simulink model "hip_controller_2026_01_27"  (R2024b)
settings: Solver=FixedStepAuto  StartTime=0.0  StopTime=simDuration  FixedStep=0.01  RelTol=1e-3  EnableMultiTasking=on
InitFcn:
  | breakp=[-1, -0.8, -0.6, -0.4, -0.2, -0.1, 0, 0.1, 0.2, 0.4, 0.6, 0.8, 1];
  | splinenew =[-1, -0.8, -0.6, -0.4, -0.2, -0.1, 0, 0, 0.005, 0.01, 0.015,0.02,0.025];
undefined symbols (not defined in the file or in its folder): Discrete, K, qbreak, Time
libraries: simulink x53, arduinolib x11, dspswit3 x9, ctrlSharedLib x2, dspfdesign x2, slpidlib x2
(part 4 of 4)

== system hip_controller_2026_01_27/Subsystem3/Right Motor Velocity/Subsystem/CAN Pack1/Subsystem/Buff 2 ==
  In1 : Inport
  Constant2 : Constant  Value=4  OutDataTypeStr=uint16
  Data Type Conversion2 : DataTypeConversion  OutDataTypeStr=uint8  SaturateOnIntegerOverflow=off  RndMeth=Floor
  Shift Arithmetic1 : ArithShift  BitShiftNumberSource=Input port  BitShiftNumber=8  BitShiftDirection=Right
      settings: InputPortMap=u0,p1
  Out1 : Outport
  wires:
  Shift Arithmetic1/1 -> Data Type Conversion2/1
  Data Type Conversion2/1 -> Out1/1
  In1/1 -> Shift Arithmetic1/1
  Constant2/1 -> Shift Arithmetic1/2

== system hip_controller_2026_01_27/Subsystem3/Right Motor Velocity/Subsystem/CAN Pack1/Subsystem/Buff 3 ==
  In1 : Inport
  In2 : Inport  Port=2
  Bitwise AND1 : simulink/Logic and Bit Operations/Bitwise Operator  logicop=AND  UseBitMask=on  BitMask=bin2dec('000000001111')  BitMaskRealWorld=Stored Integer
  Bitwise OR1 : simulink/Logic and Bit Operations/Bitwise Operator  logicop=OR  UseBitMask=off  NumInputPorts=2  BitMask=bin2dec('11011001')  BitMaskRealWorld=Stored Integer
  Constant1 : Constant  Value=8  OutDataTypeStr=uint16
  Constant2 : Constant  Value=4  OutDataTypeStr=uint16
  Data Type Conversion3 : DataTypeConversion  OutDataTypeStr=uint8  SaturateOnIntegerOverflow=off  RndMeth=Floor
  Shift Arithmetic3 : ArithShift  BitShiftNumberSource=Input port  BitShiftNumber=8  BitShiftDirection=Left
      settings: InputPortMap=u0,p1
  Shift Arithmetic4 : ArithShift  BitShiftNumberSource=Input port  BitShiftNumber=8  BitShiftDirection=Right
      settings: InputPortMap=u0,p1
  Out1 : Outport
  wires:
  Shift Arithmetic3/1 -> Bitwise OR1/1
  In1/1 -> Bitwise AND1/1
  Constant1/1 -> Shift Arithmetic4/2
  Bitwise AND1/1 -> Shift Arithmetic3/1
  Shift Arithmetic4/1 -> Bitwise OR1/2
  In2/1 -> Shift Arithmetic4/1
  Bitwise OR1/1 -> Data Type Conversion3/1
  Data Type Conversion3/1 -> Out1/1
  Constant2/1 -> Shift Arithmetic3/2

== system hip_controller_2026_01_27/Subsystem3/Right Motor Velocity/Subsystem/CAN Pack1/Subsystem/Buff 4 ==
  In1 : Inport
  Bitwise AND3 : simulink/Logic and Bit Operations/Bitwise Operator  logicop=AND  UseBitMask=on  BitMask=bin2dec('000011111111')  BitMaskRealWorld=Stored Integer
  Data Type Conversion4 : DataTypeConversion  OutDataTypeStr=uint8  SaturateOnIntegerOverflow=off  RndMeth=Floor
  Out1 : Outport
  wires:
  Data Type Conversion4/1 -> Out1/1
  Bitwise AND3/1 -> Data Type Conversion4/1
  In1/1 -> Bitwise AND3/1

== system hip_controller_2026_01_27/Subsystem3/Right Motor Velocity/Subsystem/CAN Pack1/Subsystem/Buff 5 ==
  In2 : Inport
  Constant2 : Constant  Value=4  OutDataTypeStr=uint16
  Data Type Conversion5 : DataTypeConversion  OutDataTypeStr=uint8  SaturateOnIntegerOverflow=off  RndMeth=Floor
  Shift Arithmetic5 : ArithShift  BitShiftNumberSource=Input port  BitShiftNumber=8  BitShiftDirection=Right
      settings: InputPortMap=u0,p1
  Out1 : Outport
  wires:
  In2/1 -> Shift Arithmetic5/1
  Shift Arithmetic5/1 -> Data Type Conversion5/1
  Data Type Conversion5/1 -> Out1/1
  Constant2/1 -> Shift Arithmetic5/2

== system hip_controller_2026_01_27/Subsystem3/Right Motor Velocity/Subsystem/CAN Pack1/Subsystem/Buff 6 ==
  In3 : Inport
  In4 : Inport  Port=2
  Bitwise AND2 : simulink/Logic and Bit Operations/Bitwise Operator  logicop=AND  UseBitMask=on  BitMask=bin2dec('000000001111')  BitMaskRealWorld=Stored Integer
  Bitwise OR2 : simulink/Logic and Bit Operations/Bitwise Operator  logicop=OR  UseBitMask=off  NumInputPorts=2  BitMask=bin2dec('11011001')  BitMaskRealWorld=Stored Integer
  Constant1 : Constant  Value=8  OutDataTypeStr=uint16
  Constant2 : Constant  Value=4  OutDataTypeStr=uint16
  Data Type Conversion6 : DataTypeConversion  OutDataTypeStr=uint8  SaturateOnIntegerOverflow=off  RndMeth=Floor
  Shift Arithmetic6 : ArithShift  BitShiftNumberSource=Input port  BitShiftNumber=8  BitShiftDirection=Left
      settings: InputPortMap=u0,p1
  Shift Arithmetic7 : ArithShift  BitShiftNumberSource=Input port  BitShiftNumber=8  BitShiftDirection=Right
      settings: InputPortMap=u0,p1
  Out1 : Outport
  wires:
  In4/1 -> Shift Arithmetic7/1
  Shift Arithmetic7/1 -> Bitwise OR2/2
  Shift Arithmetic6/1 -> Bitwise OR2/1
  Bitwise OR2/1 -> Data Type Conversion6/1
  In3/1 -> Bitwise AND2/1
  Bitwise AND2/1 -> Shift Arithmetic6/1
  Data Type Conversion6/1 -> Out1/1
  Constant2/1 -> Shift Arithmetic6/2
  Constant1/1 -> Shift Arithmetic7/2

== system hip_controller_2026_01_27/Subsystem3/Right Motor Velocity/Subsystem/CAN Pack1/Subsystem/Buff 7 ==
  In1 : Inport
  Bitwise AND4 : simulink/Logic and Bit Operations/Bitwise Operator  logicop=AND  UseBitMask=on  BitMask=bin2dec('000011111111')  BitMaskRealWorld=Stored Integer
  Data Type Conversion7 : DataTypeConversion  OutDataTypeStr=uint8  SaturateOnIntegerOverflow=off  RndMeth=Floor
  Out1 : Outport
  wires:
  Bitwise AND4/1 -> Data Type Conversion7/1
  Data Type Conversion7/1 -> Out1/1
  In1/1 -> Bitwise AND4/1

== system hip_controller_2026_01_27/Subsystem4/Left Motor Velocity/Subsystem/CAN Pack1/Subsystem/Buff 0 ==
  In1 : Inport
  Constant1 : Constant  Value=8  OutDataTypeStr=uint16
  Data Type Conversion : DataTypeConversion  OutDataTypeStr=uint8  SaturateOnIntegerOverflow=off  RndMeth=Floor
  Shift Arithmetic2 : ArithShift  BitShiftNumberSource=Input port  BitShiftNumber=8  BitShiftDirection=Right
      settings: InputPortMap=u0,p1
  Out1 : Outport
  wires:
  In1/1 -> Shift Arithmetic2/1
  Shift Arithmetic2/1 -> Data Type Conversion/1
  Data Type Conversion/1 -> Out1/1
  Constant1/1 -> Shift Arithmetic2/2

== system hip_controller_2026_01_27/Subsystem4/Left Motor Velocity/Subsystem/CAN Pack1/Subsystem/Buff 1 ==
  In1 : Inport
  Bitwise AND : simulink/Logic and Bit Operations/Bitwise Operator  logicop=AND  UseBitMask=on  BitMask=bin2dec('0000000011111111')  BitMaskRealWorld=Stored Integer
  Data Type Conversion1 : DataTypeConversion  OutDataTypeStr=uint8  SaturateOnIntegerOverflow=off  RndMeth=Floor
  Out1 : Outport
  wires:
  Bitwise AND/1 -> Data Type Conversion1/1
  Data Type Conversion1/1 -> Out1/1
  In1/1 -> Bitwise AND/1

== system hip_controller_2026_01_27/Subsystem4/Left Motor Velocity/Subsystem/CAN Pack1/Subsystem/Buff 2 ==
  In1 : Inport
  Constant2 : Constant  Value=4  OutDataTypeStr=uint16
  Data Type Conversion2 : DataTypeConversion  OutDataTypeStr=uint8  SaturateOnIntegerOverflow=off  RndMeth=Floor
  Shift Arithmetic1 : ArithShift  BitShiftNumberSource=Input port  BitShiftNumber=8  BitShiftDirection=Right
      settings: InputPortMap=u0,p1
  Out1 : Outport
  wires:
  Shift Arithmetic1/1 -> Data Type Conversion2/1
  Data Type Conversion2/1 -> Out1/1
  In1/1 -> Shift Arithmetic1/1
  Constant2/1 -> Shift Arithmetic1/2

== system hip_controller_2026_01_27/Subsystem4/Left Motor Velocity/Subsystem/CAN Pack1/Subsystem/Buff 3 ==
  In1 : Inport
  In2 : Inport  Port=2
  Bitwise AND1 : simulink/Logic and Bit Operations/Bitwise Operator  logicop=AND  UseBitMask=on  BitMask=bin2dec('000000001111')  BitMaskRealWorld=Stored Integer
  Bitwise OR1 : simulink/Logic and Bit Operations/Bitwise Operator  logicop=OR  UseBitMask=off  NumInputPorts=2  BitMask=bin2dec('11011001')  BitMaskRealWorld=Stored Integer
  Constant1 : Constant  Value=8  OutDataTypeStr=uint16
  Constant2 : Constant  Value=4  OutDataTypeStr=uint16
  Data Type Conversion3 : DataTypeConversion  OutDataTypeStr=uint8  SaturateOnIntegerOverflow=off  RndMeth=Floor
  Shift Arithmetic3 : ArithShift  BitShiftNumberSource=Input port  BitShiftNumber=8  BitShiftDirection=Left
      settings: InputPortMap=u0,p1
  Shift Arithmetic4 : ArithShift  BitShiftNumberSource=Input port  BitShiftNumber=8  BitShiftDirection=Right
      settings: InputPortMap=u0,p1
  Out1 : Outport
  wires:
  Shift Arithmetic3/1 -> Bitwise OR1/1
  In1/1 -> Bitwise AND1/1
  Constant1/1 -> Shift Arithmetic4/2
  Bitwise AND1/1 -> Shift Arithmetic3/1
  Shift Arithmetic4/1 -> Bitwise OR1/2
  In2/1 -> Shift Arithmetic4/1
  Bitwise OR1/1 -> Data Type Conversion3/1
  Data Type Conversion3/1 -> Out1/1
  Constant2/1 -> Shift Arithmetic3/2

== system hip_controller_2026_01_27/Subsystem4/Left Motor Velocity/Subsystem/CAN Pack1/Subsystem/Buff 4 ==
  In1 : Inport
  Bitwise AND3 : simulink/Logic and Bit Operations/Bitwise Operator  logicop=AND  UseBitMask=on  BitMask=bin2dec('000011111111')  BitMaskRealWorld=Stored Integer
  Data Type Conversion4 : DataTypeConversion  OutDataTypeStr=uint8  SaturateOnIntegerOverflow=off  RndMeth=Floor
  Out1 : Outport
  wires:
  Data Type Conversion4/1 -> Out1/1
  Bitwise AND3/1 -> Data Type Conversion4/1
  In1/1 -> Bitwise AND3/1

== system hip_controller_2026_01_27/Subsystem4/Left Motor Velocity/Subsystem/CAN Pack1/Subsystem/Buff 5 ==
  In2 : Inport
  Constant2 : Constant  Value=4  OutDataTypeStr=uint16
  Data Type Conversion5 : DataTypeConversion  OutDataTypeStr=uint8  SaturateOnIntegerOverflow=off  RndMeth=Floor
  Shift Arithmetic5 : ArithShift  BitShiftNumberSource=Input port  BitShiftNumber=8  BitShiftDirection=Right
      settings: InputPortMap=u0,p1
  Out1 : Outport
  wires:
  In2/1 -> Shift Arithmetic5/1
  Shift Arithmetic5/1 -> Data Type Conversion5/1
  Data Type Conversion5/1 -> Out1/1
  Constant2/1 -> Shift Arithmetic5/2

== system hip_controller_2026_01_27/Subsystem4/Left Motor Velocity/Subsystem/CAN Pack1/Subsystem/Buff 6 ==
  In3 : Inport
  In4 : Inport  Port=2
  Bitwise AND2 : simulink/Logic and Bit Operations/Bitwise Operator  logicop=AND  UseBitMask=on  BitMask=bin2dec('000000001111')  BitMaskRealWorld=Stored Integer
  Bitwise OR2 : simulink/Logic and Bit Operations/Bitwise Operator  logicop=OR  UseBitMask=off  NumInputPorts=2  BitMask=bin2dec('11011001')  BitMaskRealWorld=Stored Integer
  Constant1 : Constant  Value=8  OutDataTypeStr=uint16
  Constant2 : Constant  Value=4  OutDataTypeStr=uint16
  Data Type Conversion6 : DataTypeConversion  OutDataTypeStr=uint8  SaturateOnIntegerOverflow=off  RndMeth=Floor
  Shift Arithmetic6 : ArithShift  BitShiftNumberSource=Input port  BitShiftNumber=8  BitShiftDirection=Left
      settings: InputPortMap=u0,p1
  Shift Arithmetic7 : ArithShift  BitShiftNumberSource=Input port  BitShiftNumber=8  BitShiftDirection=Right
      settings: InputPortMap=u0,p1
  Out1 : Outport
  wires:
  In4/1 -> Shift Arithmetic7/1
  Shift Arithmetic7/1 -> Bitwise OR2/2
  Shift Arithmetic6/1 -> Bitwise OR2/1
  Bitwise OR2/1 -> Data Type Conversion6/1
  In3/1 -> Bitwise AND2/1
  Bitwise AND2/1 -> Shift Arithmetic6/1
  Data Type Conversion6/1 -> Out1/1
  Constant2/1 -> Shift Arithmetic6/2
  Constant1/1 -> Shift Arithmetic7/2

== system hip_controller_2026_01_27/Subsystem4/Left Motor Velocity/Subsystem/CAN Pack1/Subsystem/Buff 7 ==
  In1 : Inport
  Bitwise AND4 : simulink/Logic and Bit Operations/Bitwise Operator  logicop=AND  UseBitMask=on  BitMask=bin2dec('000011111111')  BitMaskRealWorld=Stored Integer
  Data Type Conversion7 : DataTypeConversion  OutDataTypeStr=uint8  SaturateOnIntegerOverflow=off  RndMeth=Floor
  Out1 : Outport
  wires:
  Bitwise AND4/1 -> Data Type Conversion7/1
  Data Type Conversion7/1 -> Out1/1
  In1/1 -> Bitwise AND4/1

== system hip_controller_2026_01_27/Subsystem4/Right Motor Velocity/Subsystem/CAN Pack1/Subsystem/Buff 0 ==
  In1 : Inport
  Constant1 : Constant  Value=8  OutDataTypeStr=uint16
  Data Type Conversion : DataTypeConversion  OutDataTypeStr=uint8  SaturateOnIntegerOverflow=off  RndMeth=Floor
  Shift Arithmetic2 : ArithShift  BitShiftNumberSource=Input port  BitShiftNumber=8  BitShiftDirection=Right
      settings: InputPortMap=u0,p1
  Out1 : Outport
  wires:
  In1/1 -> Shift Arithmetic2/1
  Shift Arithmetic2/1 -> Data Type Conversion/1
  Data Type Conversion/1 -> Out1/1
  Constant1/1 -> Shift Arithmetic2/2

== system hip_controller_2026_01_27/Subsystem4/Right Motor Velocity/Subsystem/CAN Pack1/Subsystem/Buff 1 ==
  In1 : Inport
  Bitwise AND : simulink/Logic and Bit Operations/Bitwise Operator  logicop=AND  UseBitMask=on  BitMask=bin2dec('0000000011111111')  BitMaskRealWorld=Stored Integer
  Data Type Conversion1 : DataTypeConversion  OutDataTypeStr=uint8  SaturateOnIntegerOverflow=off  RndMeth=Floor
  Out1 : Outport
  wires:
  Bitwise AND/1 -> Data Type Conversion1/1
  Data Type Conversion1/1 -> Out1/1
  In1/1 -> Bitwise AND/1

== system hip_controller_2026_01_27/Subsystem4/Right Motor Velocity/Subsystem/CAN Pack1/Subsystem/Buff 2 ==
  In1 : Inport
  Constant2 : Constant  Value=4  OutDataTypeStr=uint16
  Data Type Conversion2 : DataTypeConversion  OutDataTypeStr=uint8  SaturateOnIntegerOverflow=off  RndMeth=Floor
  Shift Arithmetic1 : ArithShift  BitShiftNumberSource=Input port  BitShiftNumber=8  BitShiftDirection=Right
      settings: InputPortMap=u0,p1
  Out1 : Outport
  wires:
  Shift Arithmetic1/1 -> Data Type Conversion2/1
  Data Type Conversion2/1 -> Out1/1
  In1/1 -> Shift Arithmetic1/1
  Constant2/1 -> Shift Arithmetic1/2

== system hip_controller_2026_01_27/Subsystem4/Right Motor Velocity/Subsystem/CAN Pack1/Subsystem/Buff 3 ==
  In1 : Inport
  In2 : Inport  Port=2
  Bitwise AND1 : simulink/Logic and Bit Operations/Bitwise Operator  logicop=AND  UseBitMask=on  BitMask=bin2dec('000000001111')  BitMaskRealWorld=Stored Integer
  Bitwise OR1 : simulink/Logic and Bit Operations/Bitwise Operator  logicop=OR  UseBitMask=off  NumInputPorts=2  BitMask=bin2dec('11011001')  BitMaskRealWorld=Stored Integer
  Constant1 : Constant  Value=8  OutDataTypeStr=uint16
  Constant2 : Constant  Value=4  OutDataTypeStr=uint16
  Data Type Conversion3 : DataTypeConversion  OutDataTypeStr=uint8  SaturateOnIntegerOverflow=off  RndMeth=Floor
  Shift Arithmetic3 : ArithShift  BitShiftNumberSource=Input port  BitShiftNumber=8  BitShiftDirection=Left
      settings: InputPortMap=u0,p1
  Shift Arithmetic4 : ArithShift  BitShiftNumberSource=Input port  BitShiftNumber=8  BitShiftDirection=Right
      settings: InputPortMap=u0,p1
  Out1 : Outport
  wires:
  Shift Arithmetic3/1 -> Bitwise OR1/1
  In1/1 -> Bitwise AND1/1
  Constant1/1 -> Shift Arithmetic4/2
  Bitwise AND1/1 -> Shift Arithmetic3/1
  Shift Arithmetic4/1 -> Bitwise OR1/2
  In2/1 -> Shift Arithmetic4/1
  Bitwise OR1/1 -> Data Type Conversion3/1
  Data Type Conversion3/1 -> Out1/1
  Constant2/1 -> Shift Arithmetic3/2

== system hip_controller_2026_01_27/Subsystem4/Right Motor Velocity/Subsystem/CAN Pack1/Subsystem/Buff 4 ==
  In1 : Inport
  Bitwise AND3 : simulink/Logic and Bit Operations/Bitwise Operator  logicop=AND  UseBitMask=on  BitMask=bin2dec('000011111111')  BitMaskRealWorld=Stored Integer
  Data Type Conversion4 : DataTypeConversion  OutDataTypeStr=uint8  SaturateOnIntegerOverflow=off  RndMeth=Floor
  Out1 : Outport
  wires:
  Data Type Conversion4/1 -> Out1/1
  Bitwise AND3/1 -> Data Type Conversion4/1
  In1/1 -> Bitwise AND3/1

== system hip_controller_2026_01_27/Subsystem4/Right Motor Velocity/Subsystem/CAN Pack1/Subsystem/Buff 5 ==
  In2 : Inport
  Constant2 : Constant  Value=4  OutDataTypeStr=uint16
  Data Type Conversion5 : DataTypeConversion  OutDataTypeStr=uint8  SaturateOnIntegerOverflow=off  RndMeth=Floor
  Shift Arithmetic5 : ArithShift  BitShiftNumberSource=Input port  BitShiftNumber=8  BitShiftDirection=Right
      settings: InputPortMap=u0,p1
  Out1 : Outport
  wires:
  In2/1 -> Shift Arithmetic5/1
  Shift Arithmetic5/1 -> Data Type Conversion5/1
  Data Type Conversion5/1 -> Out1/1
  Constant2/1 -> Shift Arithmetic5/2

== system hip_controller_2026_01_27/Subsystem4/Right Motor Velocity/Subsystem/CAN Pack1/Subsystem/Buff 6 ==
  In3 : Inport
  In4 : Inport  Port=2
  Bitwise AND2 : simulink/Logic and Bit Operations/Bitwise Operator  logicop=AND  UseBitMask=on  BitMask=bin2dec('000000001111')  BitMaskRealWorld=Stored Integer
  Bitwise OR2 : simulink/Logic and Bit Operations/Bitwise Operator  logicop=OR  UseBitMask=off  NumInputPorts=2  BitMask=bin2dec('11011001')  BitMaskRealWorld=Stored Integer
  Constant1 : Constant  Value=8  OutDataTypeStr=uint16
  Constant2 : Constant  Value=4  OutDataTypeStr=uint16
  Data Type Conversion6 : DataTypeConversion  OutDataTypeStr=uint8  SaturateOnIntegerOverflow=off  RndMeth=Floor
  Shift Arithmetic6 : ArithShift  BitShiftNumberSource=Input port  BitShiftNumber=8  BitShiftDirection=Left
      settings: InputPortMap=u0,p1
  Shift Arithmetic7 : ArithShift  BitShiftNumberSource=Input port  BitShiftNumber=8  BitShiftDirection=Right
      settings: InputPortMap=u0,p1
  Out1 : Outport
  wires:
  In4/1 -> Shift Arithmetic7/1
  Shift Arithmetic7/1 -> Bitwise OR2/2
  Shift Arithmetic6/1 -> Bitwise OR2/1
  Bitwise OR2/1 -> Data Type Conversion6/1
  In3/1 -> Bitwise AND2/1
  Bitwise AND2/1 -> Shift Arithmetic6/1
  Data Type Conversion6/1 -> Out1/1
  Constant2/1 -> Shift Arithmetic6/2
  Constant1/1 -> Shift Arithmetic7/2

== system hip_controller_2026_01_27/Subsystem4/Right Motor Velocity/Subsystem/CAN Pack1/Subsystem/Buff 7 ==
  In1 : Inport
  Bitwise AND4 : simulink/Logic and Bit Operations/Bitwise Operator  logicop=AND  UseBitMask=on  BitMask=bin2dec('000011111111')  BitMaskRealWorld=Stored Integer
  Data Type Conversion7 : DataTypeConversion  OutDataTypeStr=uint8  SaturateOnIntegerOverflow=off  RndMeth=Floor
  Out1 : Outport
  wires:
  Bitwise AND4/1 -> Data Type Conversion7/1
  Data Type Conversion7/1 -> Out1/1
  In1/1 -> Bitwise AND4/1

== matlab function hip_controller_2026_01_27/RIGHT_LEG1/Ref traj w// noise ==
  data: y input; x_hat output
function x_hat = kalman_filter(y)
% y: measured angle (scalar)
% x_hat: [theta_hat; theta_dot_hat]

persistent A C Q R P x
persistent initialized

Ts = 0.01; % sample time

if isempty(initialized)
    A = [1 Ts; 0 1];
    C = [1 0];

    % Tune these:
    Q = [1e-6      0;
        0      5e-3];    % more process noise on velocity state
    R = 9e-4;            % measurement noise variance (rad^2)

    P = eye(2);        % initial covariance
    x = [0; 0];        % initial state estimate
    initialized = true;
end

% Prediction
x_pred = A * x;
P_pred = A * P * A' + Q;

% Innovation
y_pred = C * x_pred;
e = y - y_pred;  % innovation

S = C * P_pred * C' + R;
K = P_pred * C' / S;  % Kalman gain (2x1)

% Update
x = x_pred + K * e;
P = (eye(2) - K * C) * P_pred;

x_hat = x;

== matlab function hip_controller_2026_01_27/LEFT LEG1/Ref traj w// noise ==
  data: y input; x_hat output
function x_hat = kalman_filter(y)
% y: measured angle (scalar)
% x_hat: [theta_hat; theta_dot_hat]

persistent A C Q R P x
persistent initialized

Ts = 0.01; % sample time

if isempty(initialized)
    A = [1 Ts; 0 1];
    C = [1 0];

    % Tune these:
    Q = [1e-6      0;
        0      5e-3];    % more process noise on velocity state
    R = 9e-4;            % measurement noise variance (rad^2)

    P = eye(2);        % initial covariance
    x = [0; 0];        % initial state estimate
    initialized = true;
end

% Prediction
x_pred = A * x;
P_pred = A * P * A' + Q;

% Innovation
y_pred = C * x_pred;
e = y - y_pred;  % innovation

S = C * P_pred * C' + R;
K = P_pred * C' / S;  % Kalman gain (2x1)

% Update
x = x_pred + K * e;
P = (eye(2) - K * C) * P_pred;

x_hat = x;

== stateflow chart hip_controller_2026_01_27/LEFT LEG1/Pos and Vel normalized/Chart ==
  settings: updateMethod=DISCRETE  sampleTime=0.01
  state Expect_Vel_Max
    entry: valid_ang_min = 1;
    during:
    valid_vel_max = 0;
    valid_vel_min = 0;
    valid_ang_max = 0;
    valid_ang_min = 0;
  state Expect_Ang_Max
    entry: valid_vel_max = 1;
    during:
    valid_vel_max = 0;
    valid_vel_min = 0;
    valid_ang_max = 0;
    valid_ang_min = 0;
  state Resync
    valid_vel_max = 0;
    valid_vel_min = 0;
    valid_ang_max = 0;
    valid_ang_min = 0;
  state Expect_Vel_Min
    entry: valid_ang_max = 1;
    during:
    valid_vel_max = 0;
    valid_vel_min = 0;
    valid_ang_max = 0;
    valid_ang_min = 0;
  state Expect_Ang_Min
    entry: valid_vel_min = 1;
    during:
    valid_vel_max = 0;
    valid_vel_min = 0;
    valid_ang_max = 0;
    valid_ang_min = 0;
  Expect_Vel_Max -> Expect_Ang_Max [order 1] : [vel_max && after(Tmin, tick) && before(Tmax, tick) && vel > 0]
  Resync -> Expect_Ang_Max [order 1] : [vel_max && vel > 0]
  Expect_Vel_Max -> Resync [order 2] : [after(Tmax, tick)]
  Expect_Ang_Max -> Resync [order 2] : [after(Tmax, tick)]
  Expect_Ang_Max -> Expect_Vel_Min [order 1] : [ang_max && after(Tmin, tick) && before(Tmax, tick) && angle > 0]
  Expect_Ang_Min -> Expect_Vel_Max [order 2] : [ang_min && after(Tmin, tick) && before(Tmax, tick) && angle < 0]
  Resync -> Expect_Vel_Max [order 3] : [ang_min && angle < 0]
  Expect_Vel_Min -> Resync [order 1] : [after(Tmax, tick)]
  (default) -> Resync : {valid_vel_max = 0;
      | valid_vel_min = 0;
      | valid_ang_max = 0;
      | valid_ang_min = 0;}
  Resync -> Expect_Vel_Min [order 4] : [ang_max && angle > 0]
  Expect_Ang_Min -> Resync [order 1] : [after(Tmax, tick)]
  Resync -> Expect_Ang_Min [order 2] : [vel_min && vel < 0]
  Expect_Vel_Min -> Expect_Ang_Min [order 2] : [vel_min && after(Tmin, tick) && before(Tmax, tick) && vel < 0]
  data: ang_max input; vel_min input; vel_max input; ang_min input; valid_vel_max output; valid_vel_min output; valid_ang_max output; valid_ang_min output; Tmin local double =0; Tmax local double =60; vel input; angle input

== stateflow chart hip_controller_2026_01_27/RIGHT_LEG1/Pos and Vel normalized/Chart ==
  settings: updateMethod=DISCRETE  sampleTime=0.01
  state Expect_Vel_Max
    entry: valid_ang_min = 1;
    during:
    valid_vel_max = 0;
    valid_vel_min = 0;
    valid_ang_max = 0;
    valid_ang_min = 0;
  state Expect_Ang_Max
    entry: valid_vel_max = 1;
    during:
    valid_vel_max = 0;
    valid_vel_min = 0;
    valid_ang_max = 0;
    valid_ang_min = 0;
  state Resync
    valid_vel_max = 0;
    valid_vel_min = 0;
    valid_ang_max = 0;
    valid_ang_min = 0;
  state Expect_Vel_Min
    entry: valid_ang_max = 1;
    during:
    valid_vel_max = 0;
    valid_vel_min = 0;
    valid_ang_max = 0;
    valid_ang_min = 0;
  state Expect_Ang_Min
    entry: valid_vel_min = 1;
    during:
    valid_vel_max = 0;
    valid_vel_min = 0;
    valid_ang_max = 0;
    valid_ang_min = 0;
  Expect_Vel_Max -> Expect_Ang_Max [order 1] : [vel_max && after(Tmin, tick) && before(Tmax, tick) && vel > 0]
  Resync -> Expect_Ang_Max [order 1] : [vel_max && vel > 0]
  Expect_Vel_Max -> Resync [order 2] : [after(Tmax, tick)]
  Expect_Ang_Max -> Resync [order 2] : [after(Tmax, tick)]
  Expect_Ang_Max -> Expect_Vel_Min [order 1] : [ang_max && after(Tmin, tick) && before(Tmax, tick) && angle > 0]
  Expect_Ang_Min -> Expect_Vel_Max [order 2] : [ang_min && after(Tmin, tick) && before(Tmax, tick) && angle < 0]
  Resync -> Expect_Vel_Max [order 3] : [ang_min && angle < 0]
  Expect_Vel_Min -> Resync [order 1] : [after(Tmax, tick)]
  (default) -> Resync : {valid_vel_max = 0;
      | valid_vel_min = 0;
      | valid_ang_max = 0;
      | valid_ang_min = 0;}
  Resync -> Expect_Vel_Min [order 4] : [ang_max && angle > 0]
  Expect_Ang_Min -> Resync [order 1] : [after(Tmax, tick)]
  Resync -> Expect_Ang_Min [order 2] : [vel_min && vel < 0]
  Expect_Vel_Min -> Expect_Ang_Min [order 2] : [vel_min && after(Tmin, tick) && before(Tmax, tick) && vel < 0]
  data: ang_max input; vel_min input; vel_max input; ang_min input; valid_vel_max output; valid_vel_min output; valid_ang_max output; valid_ang_min output; Tmin local double =0; Tmax local double =60; vel input; angle input

== stateflow chart hip_controller_2026_01_27/Subsystem3/Chart ==
  state Reset
    vel = 0;
    enablestati=0;
  state Tensioning
    enablestati = 1;
    vel = -3;
  state Stop
    vel = 0;
  state Disable
    enablestati = -1;
  (default) -> Reset
  Reset -> Tensioning : [ON_OFF == 1]
  Tensioning -> Disable [order 2] : [ON_OFF == 0]
  Tensioning -> Stop [order 1] : [MOTOR_TORQUE >= 0.85]
  Stop -> Disable : after(1,sec)
  data: MOTOR_TORQUE input; ON_OFF input; thrtorque local; enablestati output; vel output

== stateflow chart hip_controller_2026_01_27/Subsystem3/Chart1 ==
  state Reset
    vel = 0;
    enablestati=0;
  state Tensioning
    enablestati = 1;
    vel = 3;
  state Stop
    vel = 0;
  state Disable
    enablestati = -1;
  (default) -> Reset
  Reset -> Tensioning : [ON_OFF == 1]
  Tensioning -> Disable [order 2] : [ON_OFF == 0]
  Tensioning -> Stop [order 1] : [MOTOR_TORQUE >= 0.85]
  Stop -> Disable : after(1,sec)
  data: MOTOR_TORQUE input; ON_OFF input; thrtorque local; enablestati output; vel output

== matlab function hip_controller_2026_01_27/Prerecorded Data/MATLAB Function ==
  data: i input; y output; data input
function y = imuPlayback(i, data)
%#codegen
% imuData must be defined as a Simulink.Parameter in the base workspace.
% Example: imuData = Simulink.Parameter(yourIMUArray);
% y will be a 1x4 row vector
if i+1 <= size(data,1)
    y = data(i+1,:);      % pick row i
else
    y = data(end,:);    % after end, hold last value
end
end

== matlab function hip_controller_2026_01_27/MATLAB Function ==
  data: Gait_phaseR input; Gait_phaseL input; STOPR input; STOPL input; output output; MMotionR input; MMotionL input
function output= fcn(Gait_phaseR, Gait_phaseL, STOPR, STOPL, MMotionR, MMotionL)
     output = [Gait_phaseR; Gait_phaseL; STOPR; STOPL; MMotionR; MMotionL];
end
